simulink model "simulation_pwm_rectifier_new"  (R2021a)
settings: Solver=VariableStepAuto  StartTime=0.0  StopTime=0.1  RelTol=1e-3
values from neighbouring files (symbols this model uses):
  f = 50    [variables.m]
  fs = 10000    [variables.m]
  k = 1.2    [variables.m]
  Vp = 100    [variables.m]
libraries: spsMosfetLib x6, spsSeriesRLCBranchLib x5, spsCurrentMeasurementLib x4, spsVoltageMeasurementLib x4, spsACVoltageSourceLib x3, spsGroundLib x1, simulink x1, spspowerguiLib x1
settings Model: Creator=Hp  LastModifiedBy=Hp

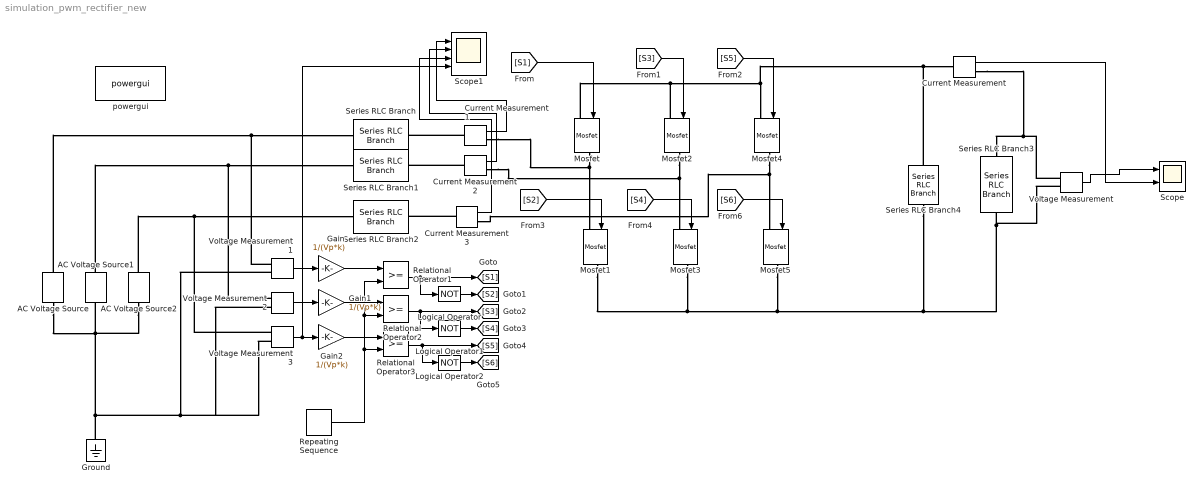
== system simulation_pwm_rectifier_new ==
  AC Voltage Source : spsACVoltageSourceLib/AC Voltage Source  Amplitude=Vp  Phase=0  Frequency=f  SampleTime=0  Measurements=None  BusType=swing  Pref=10e3  Qref=0  Qmin=-inf  Qmax=+inf
  AC Voltage Source1 : spsACVoltageSourceLib/AC Voltage Source  Amplitude=Vp  Phase=240  Frequency=f  SampleTime=0  Measurements=None  BusType=swing  Pref=10e3  Qref=0  Qmin=-inf  Qmax=+inf
  AC Voltage Source2 : spsACVoltageSourceLib/AC Voltage Source  Amplitude=Vp  Phase=120  Frequency=f  SampleTime=0  Measurements=None  BusType=swing  Pref=10e3  Qref=0  Qmin=-inf  Qmax=+inf
  Current Measurement{,1..3} (4 alike) : spsCurrentMeasurementLib/Current Measurement  PhasorSimulation=off  OutputType=Complex  PSBequivalent=0
  Gain : Gain  Gain=1/(Vp*k)
  Gain1 : Gain  Gain=1/(Vp*k)
  Gain2 : Gain  Gain=1/(Vp*k)
  Ground : spsGroundLib/Ground  LConnTagsString=a
  Logical Operator : Logic  Operator=NOT  AllPortsSameDT=off  OutDataTypeStr=boolean
  Logical Operator1 : Logic  Operator=NOT  AllPortsSameDT=off  OutDataTypeStr=boolean
  Logical Operator2 : Logic  Operator=NOT  AllPortsSameDT=off  OutDataTypeStr=boolean
  Mosfet{,1..5} (6 alike) : spsMosfetLib/Mosfet  Ron=0.1  Lon=0  Rd=0.01  Vfd=0  IC=0  Rs=1e5  Cs=inf  Measurements=off
  Relational Operator1 : RelationalOperator  OutDataTypeStr=boolean  RndMeth=Simplest
  Relational Operator2 : RelationalOperator  OutDataTypeStr=boolean  RndMeth=Simplest
  Relational Operator3 : RelationalOperator  OutDataTypeStr=boolean  RndMeth=Simplest
  Repeating Sequence : simulink/Sources/Repeating Sequence  rep_seq_t=[0 0.25/fs 0.5/fs 0.75/fs 1/fs]  rep_seq_y=[0 -1 0 1 0]
  Scope : Scope  NumInputPorts=2
  Scope1 : Scope  NumInputPorts=4
  Series RLC Branch : spsSeriesRLCBranchLib/Series RLC Branch  LConnTagsString=__new0  RConnTagsString=__new0  BranchType=RL  Resistance=0.5  Inductance=1e-3  SetiL0=off  InitialCurrent=0  Capacitance=0  Setx0=off  InitialVoltage=0  Measurements=None
  Series RLC Branch1 : spsSeriesRLCBranchLib/Series RLC Branch  LConnTagsString=__new0  RConnTagsString=__new0  BranchType=RL  Resistance=0.5  Inductance=1e-3  SetiL0=off  InitialCurrent=0  Capacitance=0  Setx0=off  InitialVoltage=0  Measurements=None
  Series RLC Branch2 : spsSeriesRLCBranchLib/Series RLC Branch  LConnTagsString=__new0  RConnTagsString=__new0  BranchType=RL  Resistance=0.5  Inductance=1e-3  SetiL0=off  InitialCurrent=0  Capacitance=0  Setx0=off  InitialVoltage=0  Measurements=None
  Series RLC Branch3 : spsSeriesRLCBranchLib/Series RLC Branch  LConnTagsString=__new0  RConnTagsString=__new0  BranchType=RL  Resistance=5  Inductance=1e-3  SetiL0=off  InitialCurrent=0  Capacitance=0  Setx0=off  InitialVoltage=0  Measurements=None
  Series RLC Branch4 : spsSeriesRLCBranchLib/Series RLC Branch  LConnTagsString=__new0  RConnTagsString=__new0  BranchType=C  Resistance=5  Inductance=1e-3  SetiL0=off  InitialCurrent=0  Capacitance=1e-3  Setx0=off  InitialVoltage=0  Measurements=None
  Voltage Measurement{,1..3} (4 alike) : spsVoltageMeasurementLib/Voltage Measurement  PhasorSimulation=off  OutputType=Complex  PSBequivalent=0
  powergui : spspowerguiLib/powergui  Priority=1  SimulationMode=Discrete  SampleTime=2e-6  frequency=60  Iterations=50  frequencyindice=50  Pbase=100e6  ErrMax=1e-4  UnitsV=kV  UnitsW=MW  buscounter=0  FunctionMessages=off  echomessages=off  EnableUseOfTLC=off  CurrentSourceSwitches=off  DisableSnubberDevices=off  DisableRonSwitches=off  DisableVfSwitches=off  DisplayEquations=off  AutomaticDiscreteSolvers=off  SolverType=Tustin/Backward Euler (TBE)  Interpol=off  ExternalGateDelay=off  methode=off  Ts=100  x0status=blocks  SPID=on  SwTol=0  HookPort=off  NonlinearTolerance=1e-4  nMaxIteration=100  ContinueOnMaxIteration=off  RestoreLinks=warning  ResistiveCurrentMeasurement=off  Frange=[0:2:500]  Ylog=off  Xlog=on  ShowGrid=off  save=off  variable=ZData  structure=0  ZoomFFT=off  StartTime=0.0  cycles=1  DisplayStyle=1  fundamental=60  FreqAxis=off  MaxFrequency=1000  frequencyindicesteady=1  RmsSteady=1  display=off
  wires:
  Voltage Measurement/1 -> Scope/1
  Voltage Measurement1/1 -> Gain/1
  Voltage Measurement2/1 -> Gain1/1
  Voltage Measurement3/1 -> Scope1/4, Gain2/1
  Gain/1 -> Relational Operator1/1
  Gain1/1 -> Relational Operator2/1
  Gain2/1 -> Relational Operator3/1
  Repeating Sequence/1 -> Relational Operator3/2, Relational Operator2/2, Relational Operator1/2
  Relational Operator1/1 -> [S1], Logical Operator/1
  Logical Operator/1 -> [S2]
  Logical Operator1/1 -> [S4]
  Relational Operator2/1 -> [S3], Logical Operator1/1
  Relational Operator3/1 -> Logical Operator2/1, [S5]
  Logical Operator2/1 -> [S6]
  Current Measurement/1 -> Scope/2
  [S1] -> Mosfet/1
  [S3] -> Mosfet2/1
  [S5] -> Mosfet4/1
  [S2] -> Mosfet1/1
  [S4] -> Mosfet3/1
  [S6] -> Mosfet5/1
  Current Measurement1/1 -> Scope1/1
  Current Measurement2/1 -> Scope1/2
  Current Measurement3/1 -> Scope1/3
  connections:
  Ground/LConn1 -- Voltage Measurement2/LConn2 -- Voltage Measurement3/LConn2 -- Voltage Measurement1/LConn2 -- AC Voltage Source/LConn1 -- AC Voltage Source2/LConn1 -- AC Voltage Source1/LConn1
  Mosfet/RConn1 -- Current Measurement1/RConn1 -- Mosfet1/LConn1
  Mosfet2/RConn1 -- Mosfet3/LConn1 -- Current Measurement2/RConn1
  Mosfet4/RConn1 -- Mosfet5/LConn1 -- Current Measurement3/RConn1
  AC Voltage Source/RConn1 -- Voltage Measurement1/LConn1 -- Series RLC Branch/LConn1
  AC Voltage Source1/RConn1 -- Voltage Measurement2/LConn1 -- Series RLC Branch1/LConn1
  AC Voltage Source2/RConn1 -- Voltage Measurement3/LConn1 -- Series RLC Branch2/LConn1
  Mosfet2/LConn1 -- Series RLC Branch4/LConn1 -- Current Measurement/LConn1 -- Mosfet4/LConn1 -- Mosfet/LConn1
  Mosfet1/RConn1 -- Mosfet3/RConn1 -- Mosfet5/RConn1 -- Series RLC Branch4/RConn1 -- Voltage Measurement/LConn2 -- Series RLC Branch3/RConn1
  Voltage Measurement/LConn1 -- Current Measurement/RConn1 -- Series RLC Branch3/LConn1
  Current Measurement1/LConn1 -- Series RLC Branch/RConn1
  Current Measurement2/LConn1 -- Series RLC Branch1/RConn1
  Current Measurement3/LConn1 -- Series RLC Branch2/RConn1
